simulink model "balance_position_SSC_robust"  (R2024b)
settings: Solver=VariableStepAuto  StartTime=0.0  StopTime=10.0  RelTol=1e-3
values from neighbouring files (symbols this model uses):
  C = Ts/(Tc+Ts)    [Simple_observer.m]
  denLPF = [Tc, Ts-Tc]    [Simple_observer.m]
  denSpeedFilter = [1,0,0,0]    [Simple_observer.m]
  Fv_prime = Fv + 2*gbox.N^2*mot.Kt*mot.Ke/mot.R*[[1 -1];[-1 1]]    [MATRIX.m]
  g = 9.81    [balrob_params.m]
  g1 = 0    [MATRIX.m]
  M11 = 2 * wheel.Iyy + 2 * gbox.N^2 * mot.rot.Iyy + ( body.m + 2 * wheel.m + 2 * mot.rot.m ) * wheel.r^2    [MATRIX.m]
  M21 = M12    [MATRIX.m]
  M22 = body.Iyy + 2 * ( 1 - gbox.N )^2 * mot.rot.Iyy + body.m * body.zb^2 + 2 * mot.rot.m * mot.rot.zb^2    [MATRIX.m]
  ms22g = 1/g    (= 0.101936799185)    [balrob_params.m]
  numLPF = [Ts]    [Simple_observer.m]
  numSpeedFilter = 1/(N*Ts)*[1,0,0,-1]    [Simple_observer.m]
  Ts = 1e-2    (= 0.01)    [balrob_params.m]
  ua2tau1 = ( 2 * gbox.N * mot.Kt / mot.R) * [1, -1]'    [MATRIX.m]
undefined symbols (not defined in the file or in its folder): body, DiscIntNeverNeededParam, drv, gbox, mot, sens, ssc_aug, wheel
settings Model: Creator=Davide Pillon  LastModifiedBy=llp

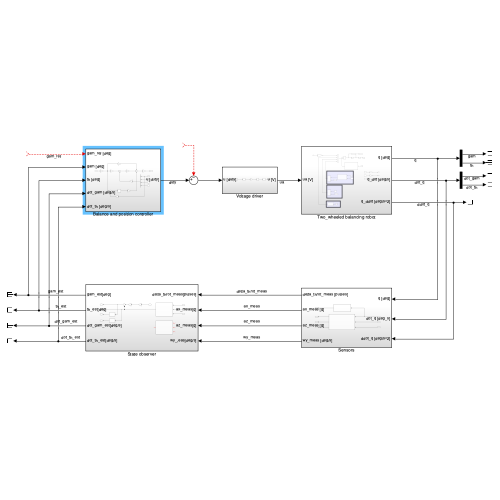
[thumbnail: Simulink's stored preview of the top-level diagram]
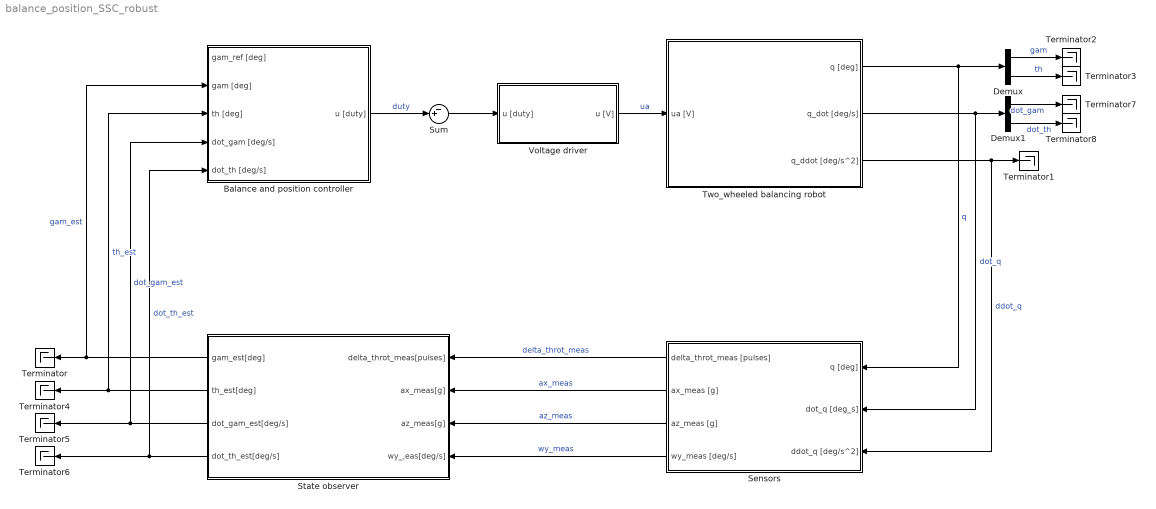
== system balance_position_SSC_robust ==
  Balance and position controller : Subsystem
  Demux : Demux  Outputs=2
  Demux1 : Demux  Outputs=2
  Sensors : Subsystem
  State observer : Subsystem
  Sum : Sum  Inputs=-+|
  Terminator{,1..8} (9 alike) : Terminator
  Two_wheeled balancing robot : Subsystem
  Voltage driver : Subsystem
  wires:
  Two_wheeled balancing robot/1(q [deg]) -> Sensors/1(q [deg]), Demux/1  "q"
  Two_wheeled balancing robot/2(q_dot [deg/s]) -> Sensors/2(dot_q [deg_s]), Demux1/1  "dot_q"
  Two_wheeled balancing robot/3(q_ddot [deg/s^2]) -> Sensors/3(ddot_q [deg/s^2]), Terminator1/1  "ddot_q"
  Demux1/1 -> Terminator7/1  "dot_gam"
  Demux1/2 -> Terminator8/1  "dot_th"
  Demux/2 -> Terminator3/1  "th"
  Demux/1 -> Terminator2/1  "gam"
  Sensors/1(delta_throt_meas [pulses]) -> State observer/1(delta_throt_meas[pulses])  "delta_throt_meas"
  Sensors/2(ax_meas [g]) -> State observer/2(ax_meas[g])  "ax_meas"
  Sensors/3(az_meas [g]) -> State observer/3(az_meas[g])  "az_meas"
  Sensors/4(wy_meas [deg/s]) -> State observer/4(wy_,eas[deg/s])  "wy_meas"
  State observer/1(gam_est[deg]) -> Balance and position controller/2(gam [deg]), Terminator/1  "gam_est"
  State observer/2(th_est[deg]) -> Balance and position controller/3(th [deg]), Terminator4/1  "th_est"
  State observer/3(dot_gam_est[deg/s]) -> Balance and position controller/4(dot_gam [deg/s]), Terminator5/1  "dot_gam_est"
  State observer/4(dot_th_est[deg/s]) -> Balance and position controller/5(dot_th [deg/s]), Terminator6/1  "dot_th_est"
  Sum/1 -> Voltage driver/1(u [duty])
  Balance and position controller/1(u [duty]) -> Sum/2  "duty"
  ? -> Sum/1
  ? -> Balance and position controller/1(gam_ref [deg])  "gam_ref"
  Voltage driver/1(u [V]) -> Two_wheeled balancing robot/1("ua [V] ")  "ua"

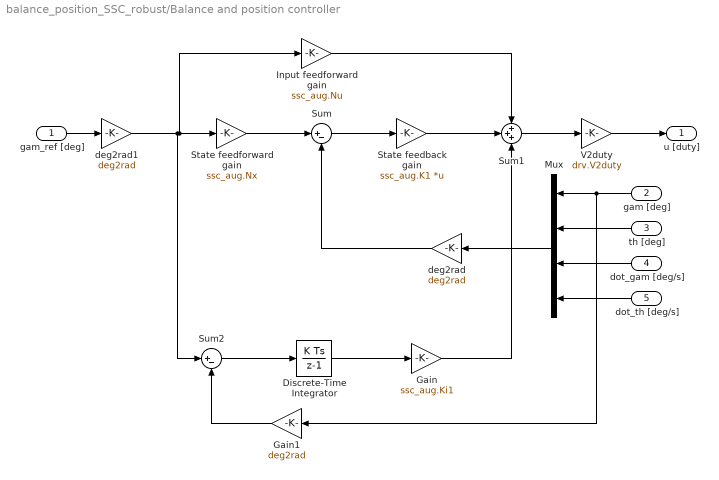
== system balance_position_SSC_robust/Balance and position controller ==
  gam_ref [deg] : Inport
  gam [deg] : Inport  Port=2
  th [deg] : Inport  Port=3
  dot_gam [deg/s] : Inport  Port=4
  dot_th [deg/s] : Inport  Port=5
  Discrete-Time Integrator : DiscreteIntegrator  SampleTime=Ts  ICPrevOutput=DiscIntNeverNeededParam  ICPrevScaledInput=DiscIntNeverNeededParam
  Gain : Gain  Gain=ssc_aug.Ki1
  Gain1 : Gain  Gain=deg2rad
  Input feedforward gain : Gain  Gain=ssc_aug.Nu
  Mux : Mux
  State feedback gain : Gain  Gain=ssc_aug.K1  Multiplication=Matrix(K*u)
  State feedforward gain : Gain  Gain=ssc_aug.Nx
  Sum : Sum  Inputs=|+-
  Sum1 : Sum  Inputs=+++
  Sum2 : Sum  Inputs=|+-
  V2duty : Gain  Gain=drv.V2duty
  deg2rad : Gain  Gain=deg2rad
  deg2rad1 : Gain  Gain=deg2rad
  u [duty] : Outport
  wires:
  Input feedforward gain/1 -> Sum1/1
  gam_ref [deg]/1 -> deg2rad1/1
  th [deg]/1 -> Mux/2
  deg2rad1/1 -> Sum2/1, Input feedforward gain/1, State feedforward gain/1
  Sum1/1 -> V2duty/1
  V2duty/1 -> u [duty]/1
  State feedback gain/1 -> Sum1/2
  Sum/1 -> State feedback gain/1
  gam [deg]/1 -> Gain1/1, Mux/1
  State feedforward gain/1 -> Sum/1
  dot_gam [deg/s]/1 -> Mux/3
  dot_th [deg/s]/1 -> Mux/4
  deg2rad/1 -> Sum/2
  Mux/1 -> deg2rad/1
  Discrete-Time Integrator/1 -> Gain/1
  Gain/1 -> Sum1/3
  Sum2/1 -> Discrete-Time Integrator/1
  Gain1/1 -> Sum2/2

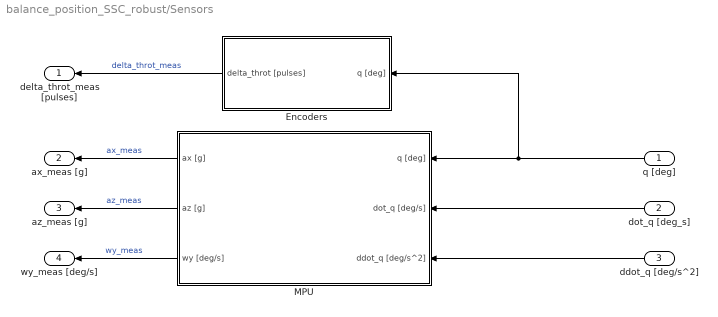
== system balance_position_SSC_robust/Sensors ==
  q [deg] : Inport
  dot_q [deg_s] : Inport  Port=2
  ddot_q [deg/s^2] : Inport  Port=3
  Encoders : Subsystem
  MPU : Subsystem
  delta_throt_meas [pulses] : Outport
  ax_meas [g] : Outport  Port=2
  az_meas [g] : Outport  Port=3
  wy_meas [deg/s] : Outport  Port=4
  wires:
  MPU/1(ax [g]) -> ax_meas [g]/1  "ax_meas"
  dot_q [deg_s]/1 -> MPU/2(dot_q [deg/s])
  MPU/2(az [g]) -> az_meas [g]/1  "az_meas"
  q [deg]/1 -> Encoders/1(q [deg]), MPU/1(q [deg])
  Encoders/1(delta_throt [pulses]) -> delta_throt_meas [pulses]/1  "delta_throt_meas"
  MPU/3(wy [deg/s]) -> wy_meas [deg/s]/1  "wy_meas"
  ddot_q [deg/s^2]/1 -> MPU/3(ddot_q [deg/s^2])

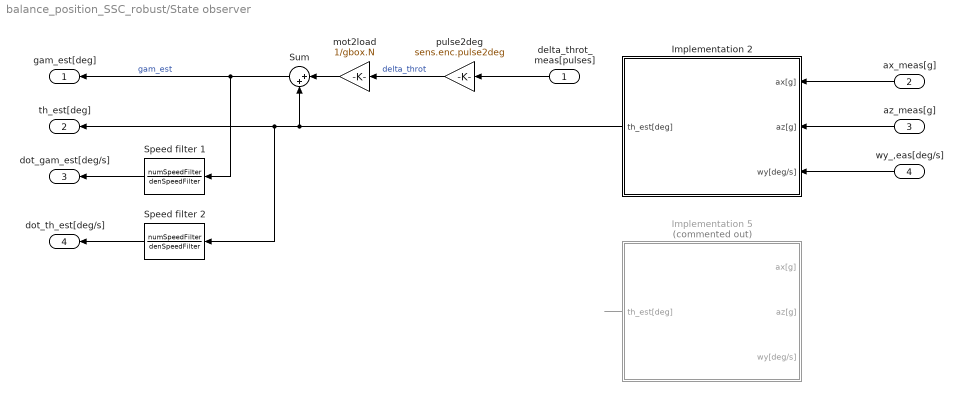
== system balance_position_SSC_robust/State observer ==
  delta_throt_meas[pulses] : Inport
  ax_meas[g] : Inport  Port=2
  az_meas[g] : Inport  Port=3
  wy_,eas[deg/s] : Inport  Port=4
  Implementation 2 : Subsystem
  Implementation 5 : Subsystem  Commented=on
  Speed filter 1 : DiscreteTransferFcn  Numerator=numSpeedFilter  Denominator=denSpeedFilter
  Speed filter 2 : DiscreteTransferFcn  Numerator=numSpeedFilter  Denominator=denSpeedFilter
  Sum : Sum  Inputs=|++
  mot2load : Gain  Gain=1/gbox.N
  pulse2deg : Gain  Gain=sens.enc.pulse2deg
  gam_est[deg] : Outport
  th_est[deg] : Outport  Port=2
  dot_gam_est[deg/s] : Outport  Port=3
  dot_th_est[deg/s] : Outport  Port=4
  wires:
  ax_meas[g]/1 -> Implementation 2/1(ax[g])
  Speed filter 2/1 -> dot_th_est[deg/s]/1
  Sum/1 -> gam_est[deg]/1, Speed filter 1/1  "gam_est"
  mot2load/1 -> Sum/1
  wy_,eas[deg/s]/1 -> Implementation 2/3(wy[deg/s])
  delta_throt_meas[pulses]/1 -> pulse2deg/1
  Implementation 2/1(th_est[deg]) -> Sum/2, th_est[deg]/1, Speed filter 2/1
  ? -> Implementation 5/2(az[g])
  az_meas[g]/1 -> Implementation 2/2(az[g])
  Speed filter 1/1 -> dot_gam_est[deg/s]/1
  pulse2deg/1 -> mot2load/1  "delta_throt"
  ? -> Implementation 5/3(wy[deg/s])
  Implementation 5/1(th_est[deg]) -> ?
  ? -> Implementation 5/1(ax[g])

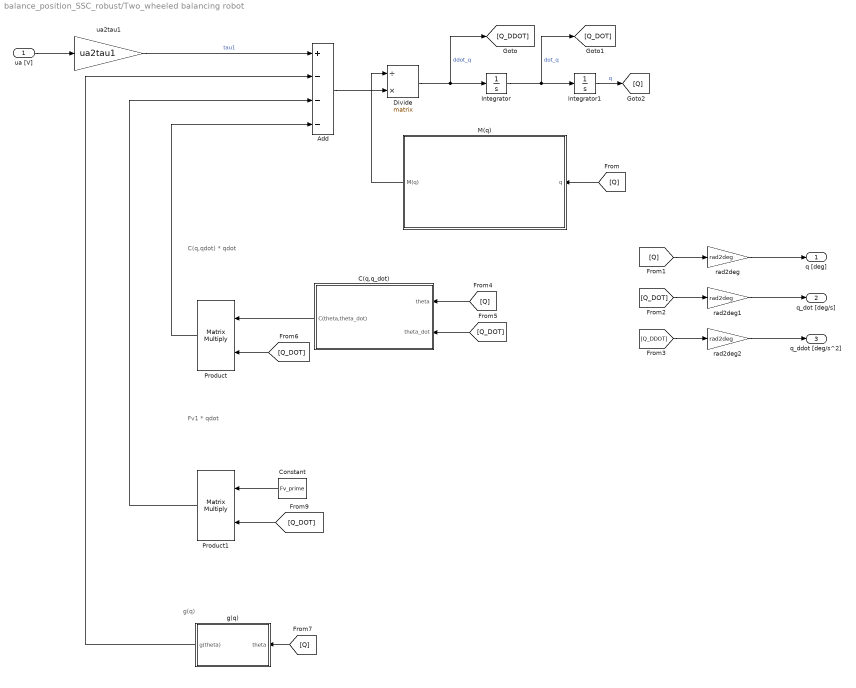
== system balance_position_SSC_robust/Two_wheeled balancing robot ==
  note: g(q)
  note: C(q,qdot) * qdot
  note: Fv1 * qdot
  "ua [V] " : Inport
  Add : Sum  Inputs=+---
  C(q,q_dot) : Subsystem
  Constant : Constant  Value=Fv_prime
  Divide : Product  Inputs=/*  Multiplication=Matrix(*)
  Integrator : Integrator
  Integrator1 : Integrator
  M(q) : Subsystem
  Product : Product  Multiplication=Matrix(*)
  Product1 : Product  Multiplication=Matrix(*)
  g(q) : Subsystem
  rad2deg : Gain  Gain=rad2deg
  rad2deg1 : Gain  Gain=rad2deg
  rad2deg2 : Gain  Gain=rad2deg
  ua2tau1 : Gain  Gain=ua2tau1
  q [deg] : Outport
  q_dot [deg/s] : Outport  Port=2
  q_ddot [deg/s^2] : Outport  Port=3
  wires:
  Constant/1 -> Product1/1
  rad2deg2/1 -> q_ddot [deg/s^2]/1
  g(q)/1(g(theta)) -> Add/2
  [Q] -> g(q)/1(theta)
  Product/1 -> Add/4
  [Q] -> C(q,q_dot)/1(theta)
  ua2tau1/1 -> Add/1  "tau1"
  [Q_DOT] -> C(q,q_dot)/2(theta_dot)
  rad2deg/1 -> q [deg]/1
  M(q)/1(M(q)) -> Divide/1
  Divide/1 -> [Q_DDOT], Integrator/1  "ddot_q"
  "ua [V] "/1 -> ua2tau1/1
  Product1/1 -> Add/3
  C(q,q_dot)/1(C(theta,theta_dot)) -> Product/1
  Add/1 -> Divide/2
  [Q_DOT] -> Product1/2
  rad2deg1/1 -> q_dot [deg/s]/1
  Integrator1/1 -> [Q]  "q"
  [Q_DOT] -> rad2deg1/1
  [Q] -> M(q)/1(q)
  Integrator/1 -> [Q_DOT], Integrator1/1  "dot_q"
  [Q_DOT] -> Product/2
  [Q] -> rad2deg/1
  [Q_DDOT] -> rad2deg2/1

== system balance_position_SSC_robust/Voltage driver ==
  u [duty] : Inport
  ZOH : ZeroOrderHold  SampleTime=Ts
  duty saturation : Saturate  UpperLimit=drv.dutymax  LowerLimit=-drv.dutymax
  duty2V : Gain  Gain=drv.duty2V
  rounding Function : Rounding  Operator=fix
  voltage saturation : Saturate  UpperLimit=drv.Vbus  LowerLimit=-drv.Vbus
  u [V] : Outport
  wires:
  duty saturation/1 -> rounding Function/1
  u [duty]/1 -> duty saturation/1
  rounding Function/1 -> duty2V/1
  voltage saturation/1 -> ZOH/1
  ZOH/1 -> u [V]/1
  duty2V/1 -> voltage saturation/1

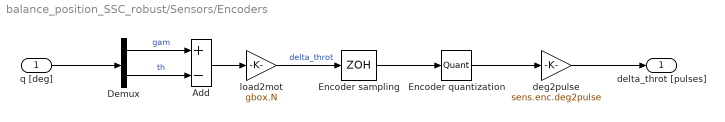
== system balance_position_SSC_robust/Sensors/Encoders ==
  q [deg] : Inport
  Add : Sum  Inputs=+-
  Demux : Demux  Outputs=2
  Encoder quantization : Quantizer  QuantizationInterval=sens.enc.pulse2deg
  Encoder sampling : ZeroOrderHold  SampleTime=Ts
  deg2pulse : Gain  Gain=sens.enc.deg2pulse
  load2mot : Gain  Gain=gbox.N
  delta_throt [pulses] : Outport
  wires:
  Encoder quantization/1 -> deg2pulse/1
  Encoder sampling/1 -> Encoder quantization/1
  Demux/2 -> Add/2  "th"
  q [deg]/1 -> Demux/1
  Demux/1 -> Add/1  "gam"
  load2mot/1 -> Encoder sampling/1  "delta_throt"
  Add/1 -> load2mot/1
  deg2pulse/1 -> delta_throt [pulses]/1

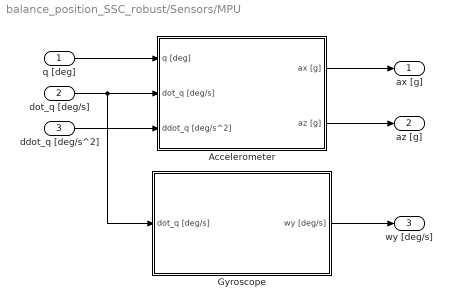
== system balance_position_SSC_robust/Sensors/MPU ==
  q [deg] : Inport
  dot_q [deg/s] : Inport  Port=2
  ddot_q [deg/s^2] : Inport  Port=3
  Accelerometer : Subsystem
  Gyroscope : Subsystem
  ax [g] : Outport
  az [g] : Outport  Port=2
  wy [deg/s] : Outport  Port=3
  wires:
  Gyroscope/1(wy [deg/s]) -> wy [deg/s]/1
  Accelerometer/1(ax [g]) -> ax [g]/1
  ddot_q [deg/s^2]/1 -> Accelerometer/3(ddot_q [deg/s^2])
  q [deg]/1 -> Accelerometer/1(q [deg])
  Accelerometer/2(az [g]) -> az [g]/1
  dot_q [deg/s]/1 -> Accelerometer/2(dot_q [deg/s]), Gyroscope/1(dot_q [deg/s])

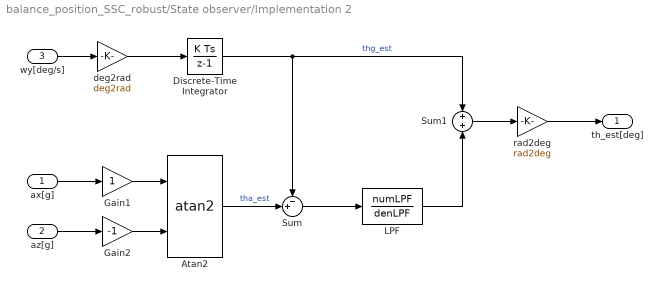
== system balance_position_SSC_robust/State observer/Implementation 2 ==
  ax[g] : Inport
  az[g] : Inport  Port=2
  wy[deg/s] : Inport  Port=3
  Atan2 : Trigonometry  Operator=atan2
  Discrete-Time Integrator : DiscreteIntegrator  SampleTime=Ts  ICPrevOutput=DiscIntNeverNeededParam  ICPrevScaledInput=DiscIntNeverNeededParam
  Gain1 : Gain
  Gain2 : Gain  Gain=-1
  LPF : DiscreteTransferFcn  Numerator=numLPF  Denominator=denLPF
  Sum : Sum  Inputs=-+|
  Sum1 : Sum
  deg2rad : Gain  Gain=deg2rad
  rad2deg : Gain  Gain=rad2deg
  th_est[deg] : Outport
  wires:
  wy[deg/s]/1 -> deg2rad/1
  ax[g]/1 -> Gain1/1
  az[g]/1 -> Gain2/1
  Gain1/1 -> Atan2/1
  Gain2/1 -> Atan2/2
  Atan2/1 -> Sum/2  "tha_est"
  deg2rad/1 -> Discrete-Time Integrator/1
  Discrete-Time Integrator/1 -> Sum1/1, Sum/1  "thg_est"
  rad2deg/1 -> th_est[deg]/1
  Sum1/1 -> rad2deg/1
  Sum/1 -> LPF/1
  LPF/1 -> Sum1/2

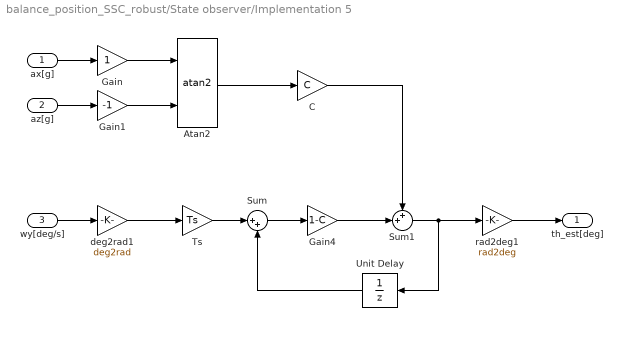
== system balance_position_SSC_robust/State observer/Implementation 5 ==
  ax[g] : Inport
  az[g] : Inport  Port=2
  wy[deg/s] : Inport  Port=3
  Atan2 : Trigonometry  Operator=atan2
  C : Gain  Gain=C
  Gain : Gain
  Gain1 : Gain  Gain=-1
  Gain4 : Gain  Gain=1-C
  Sum : Sum  Inputs=|++
  Sum1 : Sum  Inputs=++|
  Ts : Gain  Gain=Ts
  Unit Delay : UnitDelay  SampleTime=-1  HasFrameUpgradeWarning=on
  deg2rad1 : Gain  Gain=deg2rad
  rad2deg1 : Gain  Gain=rad2deg
  th_est[deg] : Outport
  wires:
  ax[g]/1 -> Gain/1
  az[g]/1 -> Gain1/1
  wy[deg/s]/1 -> deg2rad1/1
  deg2rad1/1 -> Ts/1
  Ts/1 -> Sum/1
  Sum/1 -> Gain4/1
  Unit Delay/1 -> Sum/2
  Gain4/1 -> Sum1/2
  Sum1/1 -> Unit Delay/1, rad2deg1/1
  rad2deg1/1 -> th_est[deg]/1
  Gain/1 -> Atan2/1
  Gain1/1 -> Atan2/2
  Atan2/1 -> C/1
  C/1 -> Sum1/1

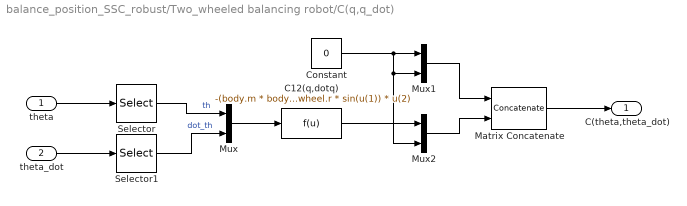
== system balance_position_SSC_robust/Two_wheeled balancing robot/C(q,q_dot) ==
  theta : Inport
  theta_dot : Inport  Port=2
  C12(q,dotq) : Fcn  Expr=-(body.m * body.zb + 2 * mot.rot.m * mot.rot.zb ) * wheel.r * sin(u(1)) * u(2)
  Constant : Constant  Value=0
  Matrix Concatenate : Concatenate  Mode=Multidimensional array  ConcatenateDimension=2
  Mux : Mux  Inputs=2
  Mux1 : Mux  Inputs=2
  Mux2 : Mux  Inputs=2
  Selector : Selector  InputPortWidth=2  IndexOptions=Index vector (dialog)  Indices=[2]  OutputSizes=1
  Selector1 : Selector  InputPortWidth=2  IndexOptions=Index vector (dialog)  Indices=[2]  OutputSizes=1
  C(theta,theta_dot) : Outport
  wires:
  Matrix Concatenate/1 -> C(theta,theta_dot)/1
  Mux2/1 -> Matrix Concatenate/2
  theta/1 -> Selector/1
  Constant/1 -> Mux2/2, Mux1/2, Mux1/1
  Mux/1 -> C12(q,dotq)/1
  Mux1/1 -> Matrix Concatenate/1
  Selector1/1 -> Mux/2  "dot_th"
  theta_dot/1 -> Selector1/1
  Selector/1 -> Mux/1  "th"
  C12(q,dotq)/1 -> Mux2/1

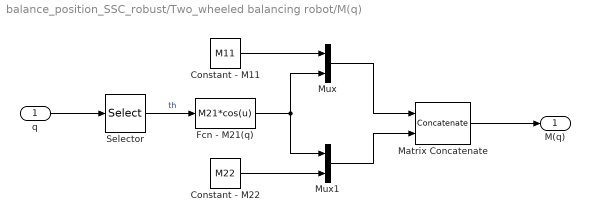
== system balance_position_SSC_robust/Two_wheeled balancing robot/M(q) ==
  q : Inport
  Constant - M11 : Constant  Value=M11
  Constant - M22 : Constant  Value=M22
  Fcn - M21(q) : Fcn  Expr=M21*cos(u)
  Matrix Concatenate : Concatenate  Mode=Multidimensional array  ConcatenateDimension=2
  Mux : Mux  Inputs=2
  Mux1 : Mux  Inputs=2
  Selector : Selector  InputPortWidth=2  IndexOptions=Index vector (dialog)  Indices=[2]  OutputSizes=1
  M(q) : Outport
  wires:
  Matrix Concatenate/1 -> M(q)/1
  Constant - M22/1 -> Mux1/2
  Fcn - M21(q)/1 -> Mux1/1, Mux/2
  q/1 -> Selector/1
  Mux/1 -> Matrix Concatenate/1
  Mux1/1 -> Matrix Concatenate/2
  Selector/1 -> Fcn - M21(q)/1  "th"
  Constant - M11/1 -> Mux/1

== system balance_position_SSC_robust/Two_wheeled balancing robot/g(q) ==
  theta : Inport
  Constant - g1 : Constant  Value=g1
  Fcn - g2(q) : Fcn  Expr=-(body.m * body.zb + 2 * mot.rot.m * mot.rot.zb) * g * sin(u)
  Mux : Mux  Inputs=2
  Selector : Selector  InputPortWidth=2  IndexOptions=Index vector (dialog)  Indices=[2]  OutputSizes=1
  g(theta) : Outport
  wires:
  Constant - g1/1 -> Mux/1
  Fcn - g2(q)/1 -> Mux/2
  Selector/1 -> Fcn - g2(q)/1  "th"
  theta/1 -> Selector/1
  Mux/1 -> g(theta)/1

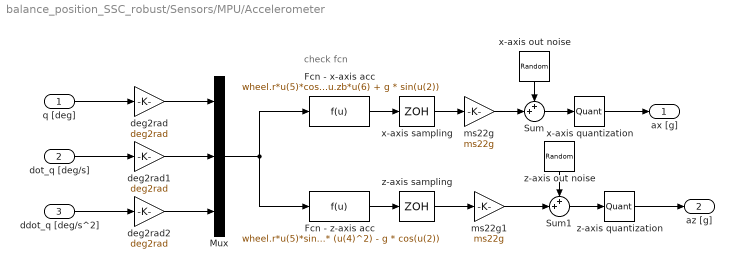
== system balance_position_SSC_robust/Sensors/MPU/Accelerometer ==
  note: check fcn
  q [deg] : Inport
  dot_q [deg/s] : Inport  Port=2
  ddot_q [deg/s^2] : Inport  Port=3
  Fcn - x-axis acc : Fcn  Expr=wheel.r*u(5)*cos(u(2)) + sens.mpu.zb*u(6) + g * sin(u(2))
  Fcn - z-axis acc : Fcn  Expr=wheel.r*u(5)*sin(u(2)) - sens.mpu.zb * (u(4)^2) - g * cos(u(2))
  Mux : Mux  Inputs=3
  Sum : Sum  Inputs=++|
  Sum1 : Sum  Inputs=++|
  deg2rad : Gain  Gain=deg2rad
  deg2rad1 : Gain  Gain=deg2rad
  deg2rad2 : Gain  Gain=deg2rad
  ms22g : Gain  Gain=ms22g
  ms22g1 : Gain  Gain=ms22g
  x-axis out noise : RandomNumber  Variance=sens.mpu.acc.noisevar  SampleTime=Ts
  x-axis quantization : Quantizer  QuantizationInterval=sens.mpu.acc.LSB2g
  x-axis sampling : ZeroOrderHold  SampleTime=Ts
  z-axis out noise : RandomNumber  Variance=sens.mpu.acc.noisevar  SampleTime=Ts
  z-axis quantization : Quantizer  QuantizationInterval=sens.mpu.acc.LSB2g
  z-axis sampling : ZeroOrderHold  SampleTime=Ts
  ax [g] : Outport
  az [g] : Outport  Port=2
  wires:
  x-axis quantization/1 -> ax [g]/1
  Fcn - z-axis acc/1 -> z-axis sampling/1
  dot_q [deg/s]/1 -> deg2rad1/1
  q [deg]/1 -> deg2rad/1
  Fcn - x-axis acc/1 -> x-axis sampling/1
  ddot_q [deg/s^2]/1 -> deg2rad2/1
  Mux/1 -> Fcn - z-axis acc/1, Fcn - x-axis acc/1
  z-axis quantization/1 -> az [g]/1
  z-axis out noise/1 -> Sum1/1
  z-axis sampling/1 -> ms22g1/1
  deg2rad1/1 -> Mux/2
  ms22g/1 -> Sum/2
  ms22g1/1 -> Sum1/2
  x-axis out noise/1 -> Sum/1
  Sum1/1 -> z-axis quantization/1
  deg2rad/1 -> Mux/1
  deg2rad2/1 -> Mux/3
  x-axis sampling/1 -> ms22g/1
  Sum/1 -> x-axis quantization/1

== system balance_position_SSC_robust/Sensors/MPU/Gyroscope ==
  dot_q [deg/s] : Inport
  "Random Number4 " : RandomNumber  Variance=sens.mpu.gyro.noisevar  SampleTime=Ts
  "Selector " : Selector  InputPortWidth=2  IndexOptions=Index vector (dialog)  Indices=2  OutputSizes=1
  "Sum4 " : Sum  Inputs=++|
  y-axis quantization : Quantizer  QuantizationInterval=sens.mpu.gyro.LSB2degs
  y-axis sampling : ZeroOrderHold  SampleTime=Ts
  wy [deg/s] : Outport
  wires:
  "Random Number4 "/1 -> "Sum4 "/1
  y-axis sampling/1 -> "Sum4 "/2
  "Sum4 "/1 -> y-axis quantization/1
  y-axis quantization/1 -> wy [deg/s]/1
  dot_q [deg/s]/1 -> "Selector "/1
  "Selector "/1 -> y-axis sampling/1
